simulink model "TEG"  (R2020a)
settings: Solver=VariableStepAuto  StartTime=0.0  StopTime=120  RelTol=1e-3
values from neighbouring files (symbols this model uses):
  delta_T = Th - Tc    (= 3.5)    [thermoelectric_gen_param1.m]
  m = 1    [thermoelectric_gen_param1.m]
  RL = (Vm^2)/Wm    (= 0.04)    [thermoelectric_gen_param1.m]
  Vm = 0.2    [thermoelectric_gen_param1.m]
  Wm = 1    [thermoelectric_gen_param1.m]
settings Model: Creator=charles  LastModifiedBy=Sumit
settings SFSimCC: CustomCodeUndefinedFunction=UseInterfaceOnly

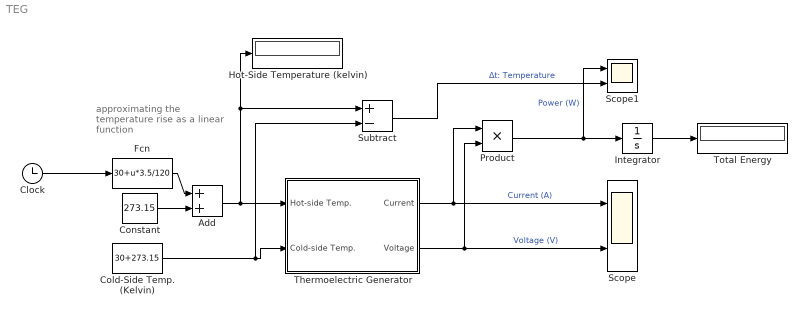
== system TEG ==
  note: approximating the temperature rise as a linear function
  Add : Sum
  Clock : Clock
  Cold-Side Temp. (Kelvin) : Constant  Value=30+273.15
  Constant : Constant  Value=273.15
  Fcn : Fcn  Expr=30+u*3.5/120
  Hot-Side Temperature (kelvin) : Display
  Integrator : Integrator
  Product : Product
  Scope : Scope  NumInputPorts=2
  Scope1 : Scope  NumInputPorts=2
  Subtract : Sum  Inputs=+-
  Thermoelectric Generator : Subsystem
  Total Energy : Display
  wires:
  Cold-Side Temp. (Kelvin)/1 -> Subtract/2, Thermoelectric Generator/2(Cold-side Temp.)
  Add/1 -> Subtract/1, Hot-Side Temperature (kelvin)/1, Thermoelectric Generator/1(Hot-side Temp.)
  Thermoelectric Generator/2(Voltage) -> Product/2, Scope/2  "Voltage (V)"
  Thermoelectric Generator/1(Current) -> Product/1, Scope/1  "Current (A)"
  Product/1 -> Integrator/1, Scope1/1  "Power (W)"
  Constant/1 -> Add/2
  Fcn/1 -> Add/1
  Subtract/1 -> Scope1/2  "Δt: Temperature"
  Clock/1 -> Fcn/1
  Integrator/1 -> Total Energy/1

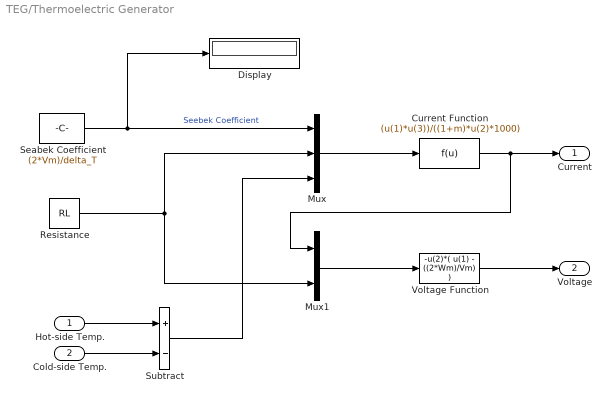
== system TEG/Thermoelectric Generator ==
  Hot-side Temp. : Inport
  Cold-side Temp. : Inport  Port=2
  Current Function : Fcn  Expr=(u(1)*u(3))/((1+m)*u(2)*1000)
  Display : Display
  Mux : Mux  Inputs=3
  Mux1 : Mux  Inputs=2
  Resistance : Constant  Value=RL
  Seabek Coefficient : Constant  Value=(2*Vm)/delta_T
  Subtract : Sum  Inputs=+-
  Voltage Function : Fcn  Expr=-u(2)*( u(1) - ((2*Wm)/Vm) )
  Current : Outport  VectorParamsAs1DForOutWhenUnconnected=off
  Voltage : Outport  Port=2  VectorParamsAs1DForOutWhenUnconnected=off
  wires:
  Hot-side Temp./1 -> Subtract/1
  Cold-side Temp./1 -> Subtract/2
  Current Function/1 -> Current/1, Mux1/1
  Mux1/1 -> Voltage Function/1
  Resistance/1 -> Mux1/2, Mux/2
  Seabek Coefficient/1 -> Display/1, Mux/1  "Seebek Coefficient"
  Voltage Function/1 -> Voltage/1
  Subtract/1 -> Mux/3
  Mux/1 -> Current Function/1
